simulink subsystem "VehicleDynamics"  (R2023b)
settings: Solver=VariableStepAuto  StartTime=0.0  StopTime=10.0  RelTol=1e-3
undefined symbols (not defined in the file): EgoCar1_params, Ts
libraries: autolibshared x1
settings Model: Creator=Victor  LastModifiedBy=victor

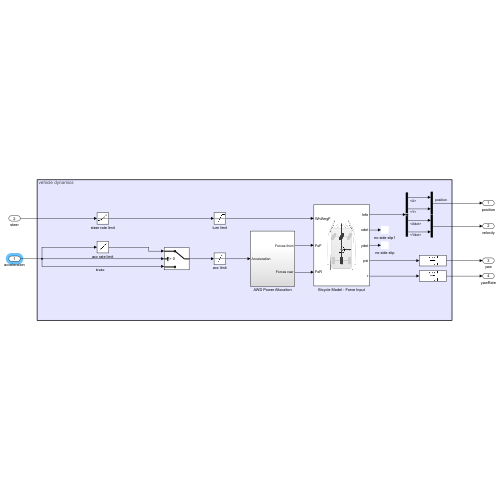
[thumbnail: Simulink's stored preview of the top-level diagram]
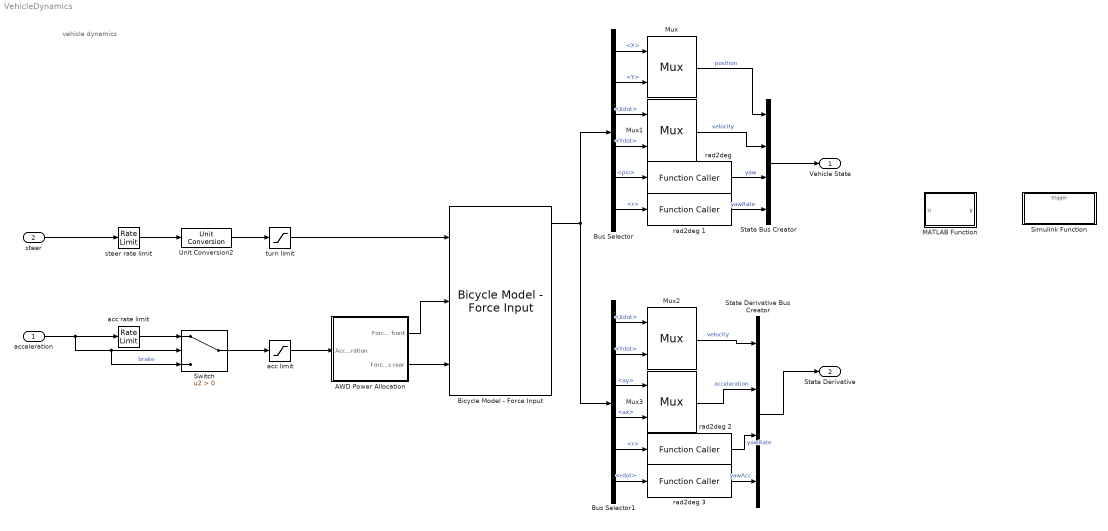
== system VehicleDynamics ==
  note: vehicle dynamics
  acceleration : Inport  Unit=m/s^2  PortDimensions=1
  steer : Inport  Port=2  Unit=deg  PortDimensions=1
  AWD Power Allocation : Subsystem
  Bicycle Model - Force Input : autolibshared/Bicycle Model - Force Input  trackMode=Single (bicycle)  inputMode=External longitudinal forces  frontSteerMode=on  rearSteerMode=off  windMode=off  muMode=off  extFMode=off  extMMode=off  aMode=3  NF=2  NR=2  m=EgoCar1_params.m  a=EgoCar1_params.lf  b=EgoCar1_params.lr  h=0.35  X_o=EgoCar1_params.state(1)  xdot_o=EgoCar1_params.state(3)  CalphaMode=off  sigmaMode=on  w=[1.4,1.4]  Cy_f=EgoCar1_params.Cf  Cy_r=EgoCar1_params.Cr  sigma_f=.1  sigma_r=.1  alpha_f_brk=[-.1 .1]  Cy_f_data=[-9e3 9e3]  alpha_r_brk=[-.1 .1]  Cy_r_data=[-9e3 9e3]  Y_o=EgoCar1_params.state(2)  ydot_o=EgoCar1_params.state(4)  Izz=EgoCar1_params.Iz  psi_o=EgoCar1_params.state(5)  r_o=EgoCar1_params.state(6)  Af=0  Cd=.3  Cl=.1  Cpm=.1  beta_w=[0:0.01:0.3]  Cs=[0:0.03:0.9]  Cym=[0:0.01:0.3]  Pabs=101325  Tair=273  g=9.81  mu=1  xdot_tol=.01  Fznom=5000  Fxtire_sat=1e6  Fytire_sat=1e6  longOff=0  latOff=0  vertOff=0
      settings: LibrarySourceBlock=drivingscenarioandsensors/Bicycle Model - Force Input
  Bus Selector : BusSelector  OutputSignals=InertFrm.Cg.Disp.X,InertFrm.Cg.Disp.Y,InertFrm.Cg.Vel.Xdot,InertFrm.Cg.Vel.Ydot,InertFrm.Cg.Ang.psi,BdyFrm.Cg.AngVel.r
  Bus Selector1 : BusSelector  OutputSignals=InertFrm.Cg.Vel.Xdot,InertFrm.Cg.Vel.Ydot,BdyFrm.Cg.Acc.ay,BdyFrm.Cg.Acc.ax,BdyFrm.Cg.AngVel.r,BdyFrm.Cg.AngAcc.rdot
  MATLAB Function : MATLAB Function  TreatAsAtomicUnit=on
  Mux{,1..3} (4 alike) : Mux  Inputs=2
      settings: DisplayOption=signals
  Simulink Function : Subsystem  TreatAsAtomicUnit=on
  State Bus Creator : BusCreator  Inputs=4
  State Derivative Bus Creator : BusCreator  Inputs=4
  Switch : Switch  Criteria=u2 > Threshold  SaturateOnIntegerOverflow=off  InputSameDT=off
  Unit Conversion2 : UnitConversion  OutputType=Inherit: Inherit via back propagation
  acc limit : Saturate  UpperLimit=EgoCar1_params.accMAX  LowerLimit=-EgoCar1_params.brakeMAX
  acc rate limit : RateLimiter  RisingSlewLimit=EgoCar1_params.jerkMAX  FallingSlewLimit=-EgoCar1_params.jerkMAX  SampleTimeMode=inherited
  rad2deg {,1..3} (4 alike) : FunctionCaller  FunctionPrototype=y = rad2deg(u)  InputArgumentSpecifications=1  OutputArgumentSpecifications=1
  steer rate limit : RateLimiter  RisingSlewLimit=EgoCar1_params.turnAngleRateMAX  FallingSlewLimit=-EgoCar1_params.turnAngleRateMAX  SampleTimeMode=inherited
  turn limit : Saturate  UpperLimit=EgoCar1_params.turnAngleMAX  LowerLimit=-EgoCar1_params.turnAngleMAX
  Vehicle State : Outport  SampleTime=Ts
  State Derivative : Outport  Port=2  SampleTime=Ts
  wires:
  "rad2deg "/1 -> State Bus Creator/3  "yaw"
  rad2deg 1/1 -> State Bus Creator/4  "yawRate"
  acc rate limit/1 -> Switch/1
  steer/1 -> steer rate limit/1
  turn limit/1 -> Bicycle Model - Force Input/1
  Switch/1 -> acc limit/1
  acc limit/1 -> AWD Power Allocation/1(Acceleration)
  AWD Power Allocation/2(Forces rear) -> Bicycle Model - Force Input/3
  acceleration/1 -> acc rate limit/1, Switch/3, Switch/2  "brake"
  AWD Power Allocation/1(Forces front) -> Bicycle Model - Force Input/2
  steer rate limit/1 -> Unit Conversion2/1
  Unit Conversion2/1 -> turn limit/1
  Mux/1 -> State Bus Creator/1  "position"
  Bus Selector/2 -> Mux/2  "<Y>"
  Bus Selector/1 -> Mux/1  "<X>"
  Bicycle Model - Force Input/1 -> Bus Selector/1, Bus Selector1/1
  Mux1/1 -> State Bus Creator/2  "velocity"
  State Bus Creator/1 -> Vehicle State/1
  Bus Selector/3 -> Mux1/1  "<Xdot>"
  Bus Selector/4 -> Mux1/2  "<Ydot>"
  Bus Selector/5 -> "rad2deg "/1  "<psi>"
  Bus Selector/6 -> rad2deg 1/1  "<r>"
  rad2deg 2/1 -> State Derivative Bus Creator/3  "yawRate"
  rad2deg 3/1 -> State Derivative Bus Creator/4  "yawAcc"
  Bus Selector1/1 -> Mux2/1  "<Xdot>"
  Mux3/1 -> State Derivative Bus Creator/2  "acceleration"
  State Derivative Bus Creator/1 -> State Derivative/1
  Bus Selector1/2 -> Mux2/2  "<Ydot>"
  Mux2/1 -> State Derivative Bus Creator/1  "velocity"
  Bus Selector1/3 -> Mux3/1  "<ay>"
  Bus Selector1/4 -> Mux3/2  "<ax>"
  Bus Selector1/5 -> rad2deg 2/1  "<r>"
  Bus Selector1/6 -> rad2deg 3/1  "<rdot>"

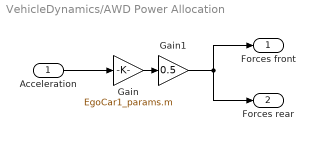
== system VehicleDynamics/AWD Power Allocation ==
  Acceleration : Inport
  Gain : Gain  Gain=EgoCar1_params.m
  Gain1 : Gain  Gain=0.5
  Forces front : Outport  VectorParamsAs1DForOutWhenUnconnected=off
  Forces rear : Outport  Port=2  VectorParamsAs1DForOutWhenUnconnected=off
  wires:
  Gain/1 -> Gain1/1
  Gain1/1 -> Forces front/1, Forces rear/1
  Acceleration/1 -> Gain/1

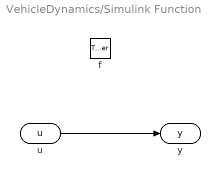
== system VehicleDynamics/Simulink Function ==
  f : TriggerPort  TriggerType=function-call  IsSimulinkFunction=on  FunctionName=f  FunctionVisibility=scoped  VariantControl=(inherit)
  u : ArgIn  DisableCoverage=on  ArgumentName=u
  y : ArgOut  DisableCoverage=on  ArgumentName=y
  wires:
  u/1 -> y/1

== matlab function VehicleDynamics/MATLAB Function ==
  data: u input; y output
function y = fcn(u)

y = u;
